simulink model "mock2dev_multidimarrays"  (R2017b)
settings: Solver=FixedStepAuto  StartTime=0.0  StopTime=10.0  FixedStep=1  RelTol=1e-3
libraries: lib_ed247 x1
settings Model: Creator=odufour  LastModifiedBy=odufour
settings DataIOCC: InspectSignalLogs=on
settings CodeAppCC: StateflowObjectComments=on

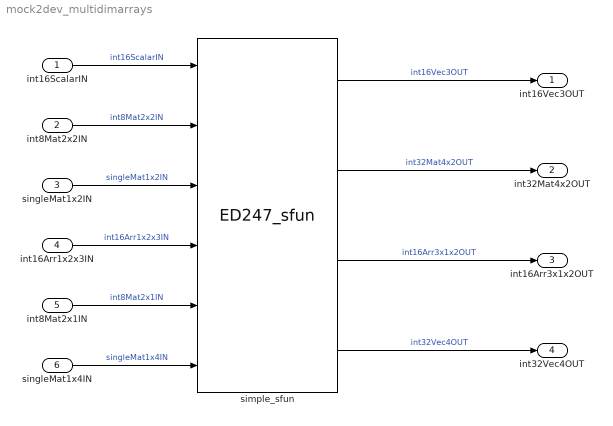
== system mock2dev_multidimarrays ==
  int16ScalarIN : Inport
  int8Mat2x2IN : Inport  Port=2
  singleMat1x2IN : Inport  Port=3
  int16Arr1x2x3IN : Inport  Port=4
  int8Mat2x1IN : Inport  Port=5
  singleMat1x4IN : Inport  Port=6
  simple_sfun : lib_ed247/ED247_sfun  configurationFilename='a429_uc_1_simple.xml'  enableLog=off  logFilename=''
      settings: SourceProductName=Airbus ED247
  int16Vec3OUT : Outport
  int32Mat4x2OUT : Outport  Port=2
  int16Arr3x1x2OUT : Outport  Port=3
  int32Vec4OUT : Outport  Port=4
  wires:
  simple_sfun/1 -> int16Vec3OUT/1  "int16Vec3OUT"
  int16ScalarIN/1 -> simple_sfun/1  "int16ScalarIN"
  int8Mat2x2IN/1 -> simple_sfun/2  "int8Mat2x2IN"
  singleMat1x2IN/1 -> simple_sfun/3  "singleMat1x2IN"
  int16Arr1x2x3IN/1 -> simple_sfun/4  "int16Arr1x2x3IN"
  int8Mat2x1IN/1 -> simple_sfun/5  "int8Mat2x1IN"
  singleMat1x4IN/1 -> simple_sfun/6  "singleMat1x4IN"
  simple_sfun/4 -> int32Vec4OUT/1  "int32Vec4OUT"
  simple_sfun/3 -> int16Arr3x1x2OUT/1  "int16Arr3x1x2OUT"
  simple_sfun/2 -> int32Mat4x2OUT/1  "int32Mat4x2OUT"
